simulink model "PMSGRectifiedBlockWindEq"  (R2022a)
settings: Solver=FixedStepDiscrete  StartTime=0.0  StopTime=65  FixedStep=20e-6  RelTol=1e-7
values from neighbouring files (symbols this model uses):
  breakpoints1 = cp_data(2:end,1)'    [FullCodePMSGDataBergy.m]
  breakpoints2 = cp_data(1,2:end)    [FullCodePMSGDataBergy.m]
  RPM_Wind_table_data = cp_data(2:end,2:end)    [FullCodePMSGDataBergy.m]
  Ts = Ts_Power    (= 2e-05)    [FullCodePMSGDataBergy.m]
  Windspeed = 11    [FullCodePMSGDataBergy.m]
  wn = (2*pi*N/60)    (= 14.6607657168)    [FullCodePMSGDataBergy.m]
libraries: spsSeriesRLCBranchLib x5, spsVoltageMeasurementLib x4, spsCurrentMeasurementLib x2, spsGroundLib x1, spsPLLLib x1, spsPermanentMagnetSynchronousMachineLib x1, spsUniversalBridgeLib x1, spspowerguiLib x1
settings Model: Creator=glopezc  LastModifiedBy=cheog

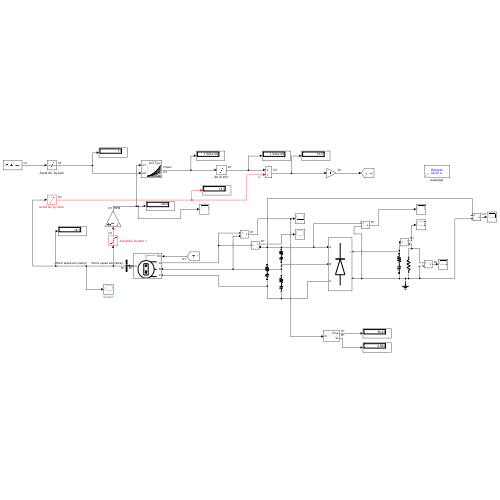
[thumbnail: Simulink's stored preview of the top-level diagram]
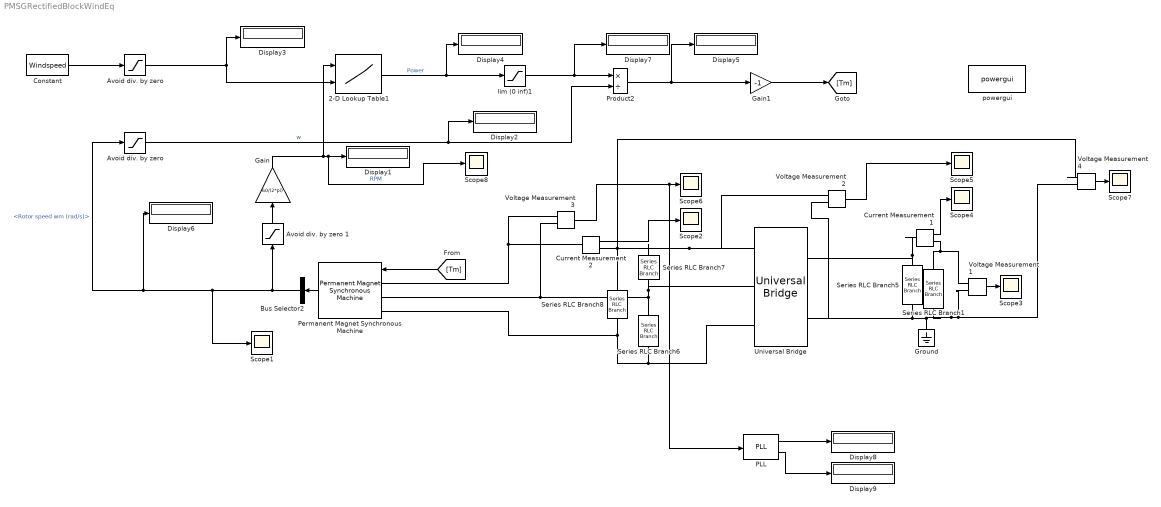
== system PMSGRectifiedBlockWindEq ==
  2-D Lookup Table1 : Lookup_n-D  BreakpointsForDimension1=breakpoints1  BreakpointsForDimension2=breakpoints2  BreakpointsForDimension1DataTypeStr=double  BreakpointsForDimension2DataTypeStr=double  Table=RPM_Wind_table_data  InternalRulePriority=Speed  OutDataTypeStr=double  RndMeth=Simplest
      settings: InputPortMap=u0,u1
  Avoid div. by zero : Saturate  UpperLimit=inf  LowerLimit=eps
  "Avoid div. by zero " : Saturate  UpperLimit=inf  LowerLimit=eps
  Avoid div. by zero 1 : Saturate  UpperLimit=inf  LowerLimit=eps
  Bus Selector2 : BusSelector  OutputSignals=Rotor speed wm (rad/s)
  Constant : Constant  Value=Windspeed
  Current Measurement1 : spsCurrentMeasurementLib/Current Measurement  PhasorSimulation=off  OutputType=Complex  PSBequivalent=0
  Current Measurement2 : spsCurrentMeasurementLib/Current Measurement  PhasorSimulation=off  OutputType=Complex  PSBequivalent=0
  Display{1..9} (9 alike) : Display
  Gain : Gain  Gain=60/(2*pi)
  Gain1 : Gain  Gain=-1
  Ground : spsGroundLib/Ground  LConnTagsString=a
  PLL : spsPLLLib/PLL  Fmin=16  Par_Init=[0, 60]  ParK=[180, 3200, 1]  TcD=1e-4  MaxRateChangeFreq=12  FilterCutOffFreq=25  Ts=Ts  AGC=on
      settings: SourceProductBaseCode=PS
  Permanent Magnet Synchronous Machine : spsPermanentMagnetSynchronousMachineLib/Permanent Magnet Synchronous Machine  NbPhases=3  FluxDistribution=Sinusoidal  RotorType=Salient-pole  MechanicalLoad=Torque Tm  PresetModel=No  ShowDetailedParameters=on  MeasurementBus=off  Resistance=0.51  Inductance=8.5e-3  dqInductances=[0.0128 0.0128]  La=0.0128  MachineConstant=Voltage Constant (V_peak L-L / krpm)  Flux=1.5637  VoltageCst=4537.9809  TorqueCst=37.5288  Flat=120  Mechanical=[174.8 0 16]  PolePairs=4  InitialConditions=[wn,0, 0,0]  InitialConditions5ph=[0 0 0 0 0 0]  RefAngle=90 degrees behind phase A axis (modified Park)  IterativeDiscreteModel=Trapezoidal non iterative  TsBlock=-1  TsPowergui=0
  Product2 : Product  Inputs=*/  InputSameDT=on  SaturateOnIntegerOverflow=on  OutDataTypeStr=Inherit: Same as first input
  Scope{1..8} (8 alike) : Scope
  Series RLC Branch1 : spsSeriesRLCBranchLib/Series RLC Branch  LConnTagsString=__new0  RConnTagsString=__new0  BranchType=R  Resistance=27.8  Inductance=1e-3  SetiL0=off  InitialCurrent=0  Capacitance=2200e-6  Setx0=off  InitialVoltage=0  Measurements=None
  Series RLC Branch5 : spsSeriesRLCBranchLib/Series RLC Branch  LConnTagsString=__new0  RConnTagsString=__new0  BranchType=RC  Resistance=.00084  Inductance=1e-3  SetiL0=off  InitialCurrent=0  Capacitance=2200e-6  Setx0=off  InitialVoltage=0  Measurements=None
  Series RLC Branch6 : spsSeriesRLCBranchLib/Series RLC Branch  LConnTagsString=__new0  RConnTagsString=__new0  BranchType=RC  Resistance=0.001  Inductance=1e-3  SetiL0=off  InitialCurrent=0  Capacitance=55e-6  Setx0=off  InitialVoltage=0  Measurements=None
  Series RLC Branch7 : spsSeriesRLCBranchLib/Series RLC Branch  LConnTagsString=__new0  RConnTagsString=__new0  BranchType=RC  Resistance=0.001  Inductance=1e-3  SetiL0=off  InitialCurrent=0  Capacitance=55e-6  Setx0=off  InitialVoltage=0  Measurements=None
  Series RLC Branch8 : spsSeriesRLCBranchLib/Series RLC Branch  LConnTagsString=__new0  RConnTagsString=__new0  BranchType=RC  Resistance=0.001  Inductance=1e-3  SetiL0=off  InitialCurrent=0  Capacitance=55e-6  Setx0=off  InitialVoltage=0  Measurements=None
  Universal Bridge : spsUniversalBridgeLib/Universal Bridge  Arms=3  SnubberResistance=Rs  SnubberCapacitance=Cs  Device=Diodes  Ron=1e-2  Lon=0  ForwardVoltages="[  0  0  ]"  ForwardVoltage=0.6  GTOparameters=[ 10e-6 , 20e-6 ]  IGBTparameters=[ 1e-6 , 2e-6 ]  Measurements=Device currents  Measurements_2=None  converterType=Rectifier
  Voltage Measurement{1..4} (4 alike) : spsVoltageMeasurementLib/Voltage Measurement  PhasorSimulation=off  OutputType=Complex  PSBequivalent=0
  lim (0 inf)1 : Saturate  UpperLimit=inf  LowerLimit=eps
  powergui : spspowerguiLib/powergui  Priority=1  SimulationMode=Discrete  SampleTime=20e-6  frequency=60  Iterations=50  frequencyindice=0  Pbase=100e6  ErrMax=1e-4  UnitsV=kV  UnitsW=MW  buscounter=0  FunctionMessages=off  echomessages=off  EnableUseOfTLC=off  CurrentSourceSwitches=off  DisableSnubberDevices=off  DisableRonSwitches=off  DisableVfSwitches=off  DisplayEquations=off  AutomaticDiscreteSolvers=off  SolverType=Tustin/Backward Euler (TBE)  Interpol=off  ExternalGateDelay=off  methode=off  Ts=100  x0status=blocks  SPID=on  SwTol=0  HookPort=off  NonlinearTolerance=1e-7  nMaxIteration=150  ContinueOnMaxIteration=off  RestoreLinks=warning  ResistiveCurrentMeasurement=off  Frange=[0:2:500]  Ylog=off  Xlog=on  ShowGrid=off  save=off  variable=ZData  structure=0  ZoomFFT=off  StartTime=0.0  cycles=1  DisplayStyle=1  fundamental=60  FreqAxis=off  MaxFrequency=1000  frequencyindicesteady=1  RmsSteady=1  display=off
  wires:
  Current Measurement1/1 -> Scope4/1
  Voltage Measurement1/1 -> Scope3/1
  Voltage Measurement3/1 -> PLL/1, Scope6/1
  Voltage Measurement4/1 -> Scope7/1
  lim (0 inf)1/1 -> Display7/1, Product2/1
  Constant/1 -> Avoid div. by zero/1
  2-D Lookup Table1/1 -> Display4/1, lim (0 inf)1/1  "Power"
  Bus Selector2/1 -> Scope1/1, Display6/1, "Avoid div. by zero "/1, Avoid div. by zero 1/1  "<Rotor speed wm (rad/s)>"
  Avoid div. by zero/1 -> 2-D Lookup Table1/2, Display3/1
  Gain/1 -> 2-D Lookup Table1/1, Scope8/1, Display1/1  "RPM"
  [Tm] -> Permanent Magnet Synchronous Machine/1
  Permanent Magnet Synchronous Machine/1 -> Bus Selector2/1
  Avoid div. by zero 1/1 -> Gain/1
  "Avoid div. by zero "/1 -> Product2/2, Display2/1  "w"
  Product2/1 -> Gain1/1, Display5/1
  Gain1/1 -> [Tm]
  Current Measurement2/1 -> Scope2/1
  Voltage Measurement2/1 -> Scope5/1
  PLL/1 -> Display8/1
  PLL/2 -> Display9/1
  connections:
  Series RLC Branch6/RConn1 -- Universal Bridge/LConn3 -- Permanent Magnet Synchronous Machine/LConn3 -- Series RLC Branch8/RConn1
  Series RLC Branch7/RConn1 -- Series RLC Branch6/LConn1 -- Permanent Magnet Synchronous Machine/LConn2 -- Voltage Measurement3/LConn2 -- Universal Bridge/LConn2
  Voltage Measurement4/LConn2 -- Ground/LConn1 -- Voltage Measurement2/LConn2 -- Universal Bridge/RConn2 -- Series RLC Branch5/RConn1 -- Series RLC Branch1/RConn1 -- Voltage Measurement1/LConn2
  Voltage Measurement1/LConn1 -- Series RLC Branch1/LConn1 -- Current Measurement1/RConn1
  Series RLC Branch5/LConn1 -- Universal Bridge/RConn1 -- Current Measurement1/LConn1
  Voltage Measurement2/LConn1 -- Universal Bridge/LConn1 -- Series RLC Branch7/LConn1 -- Current Measurement2/RConn1 -- Voltage Measurement4/LConn1 -- Series RLC Branch8/LConn1
  Voltage Measurement3/LConn1 -- Current Measurement2/LConn1 -- Permanent Magnet Synchronous Machine/LConn1
